simulink model "Test_Byte_Multiplexer_4_to_1"  (Simulink 8.7)
settings: Solver=ode45  StartTime=0.0  StopTime=len  RelTol=1e-3
libraries: Miscellaneous x5, Byte_Multiplexers_Lib x1, commutil2 x1
settings Model: Creator=N  LastModifiedBy=Jozko Mrkvicka
settings DataIOCC: LimitDataPoints=off
settings DebuggingCC: UnderspecifiedInitializationDetection=Simplified  MergeDetectMultiDrivingBlocksExec=error
settings HardwareCC: ProdBitPerPointer=64  ProdLargestAtomicFloat=Float  ProdIntDivRoundTo=Zero  ProdEndianess=LittleEndian  ProdHWDeviceType=Intel->x86-64 (Windows64)
settings ModelReferenceCC: PropagateSignalLabelsOutOfModel=on

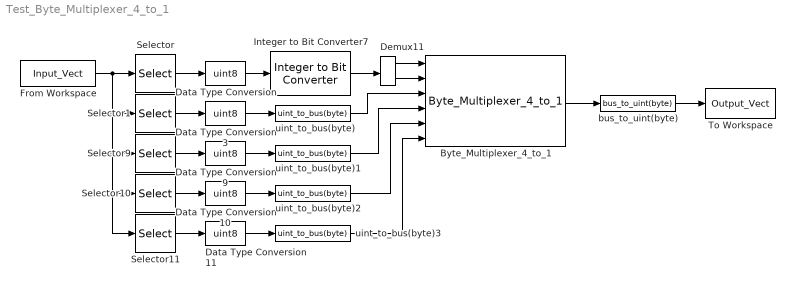
== system Test_Byte_Multiplexer_4_to_1 ==
  Byte_Multiplexer_4_to_1 : Byte_Multiplexers_Lib/Byte_Multiplexers_Lib/Byte_Multiplexer_4_to_1
  Data Type Conversion{,3,9..11} (5 alike) : DataTypeConversion  OutDataTypeStr=uint8
  Demux11 : Demux  Outputs=2
  From Workspace : FromWorkspace  VariableName=Input_Vect  SampleTime=1  Interpolate=off  OutputAfterFinalValue=Holding final value
  Integer to Bit Converter7 : commutil2/Integer to Bit Converter  nbits=2  signedInputValues=Unsigned  bitOrder=MSB first  outDtype=boolean
  Selector : Selector  IndexMode=Zero-based  InputPortWidth=5  SampleTime=1  IndexOptions=Index vector (dialog)  Indices=0  OutputSizes=1
  Selector1 : Selector  IndexMode=Zero-based  InputPortWidth=5  IndexOptions=Index vector (dialog)  Indices=1  OutputSizes=1
  Selector10 : Selector  IndexMode=Zero-based  InputPortWidth=5  IndexOptions=Index vector (dialog)  Indices=3  OutputSizes=1
  Selector11 : Selector  IndexMode=Zero-based  InputPortWidth=5  IndexOptions=Index vector (dialog)  Indices=4  OutputSizes=1
  Selector9 : Selector  IndexMode=Zero-based  InputPortWidth=5  IndexOptions=Index vector (dialog)  Indices=2  OutputSizes=1
  To Workspace : ToWorkspace  VariableName=Output_Vect  SampleTime=1
  bus_to_uint(byte) : Miscellaneous/bus_to_uint(byte)
  uint_to_bus(byte){,1..3} (4 alike) : Miscellaneous/uint_to_bus(byte)
  wires:
  Byte_Multiplexer_4_to_1/1 -> bus_to_uint(byte)/1
  Demux11/2 -> Byte_Multiplexer_4_to_1/2
  Integer to Bit Converter7/1 -> Demux11/1
  Demux11/1 -> Byte_Multiplexer_4_to_1/1
  Selector/1 -> Data Type Conversion/1
  Selector1/1 -> Data Type Conversion3/1
  Data Type Conversion3/1 -> uint_to_bus(byte)/1
  Data Type Conversion/1 -> Integer to Bit Converter7/1
  Selector9/1 -> Data Type Conversion9/1
  From Workspace/1 -> Selector11/1, Selector10/1, Selector9/1, Selector1/1, Selector/1
  Selector10/1 -> Data Type Conversion10/1
  Selector11/1 -> Data Type Conversion11/1
  Data Type Conversion9/1 -> uint_to_bus(byte)1/1
  Data Type Conversion10/1 -> uint_to_bus(byte)2/1
  Data Type Conversion11/1 -> uint_to_bus(byte)3/1
  uint_to_bus(byte)/1 -> Byte_Multiplexer_4_to_1/3
  uint_to_bus(byte)1/1 -> Byte_Multiplexer_4_to_1/4
  uint_to_bus(byte)2/1 -> Byte_Multiplexer_4_to_1/5
  uint_to_bus(byte)3/1 -> Byte_Multiplexer_4_to_1/6
  bus_to_uint(byte)/1 -> To Workspace/1
